simulink library "lib_transmission"  (Simulink 4.1.1)
undefined symbols (not defined in the file or in its folder): fc_map_spd, fc_max_trq, fc_spd_scale, fc_trq_scale, fd_inertia, fd_loss, fd_ratio, gb_inertia, gb_loss_const, gb_loss_input_spd_coeff, gb_loss_input_trq_coeff, gb_loss_output_spd_coeff, gb_loss_output_trq_coeff, gb_map_spd_out, gb_map_trq_in, gb_map_trq_out, gb_ratio, gb_spd_scale, gb_trq_scale, htc_inertia, htc_k_adv, htc_k_adv_coast, htc_max_coast_tr, htc_min_coast_tr, htc_sr, htc_sr_coast, htc_tr, htc_tr_coast, mc_map_spd, mc_max_trq, mc_overtrq_factor, mc_spd_scale, mc_trq_scale, tc_loss, tc_mc_to_fc_ratio, tx_eff_map, tx_map_spd, tx_map_trq, tx_pg_r, tx_pg_s, vc_idle_spd, vc_launch_spd
libraries: lib_transmission x2
(part 3 of 3)

== system lib_transmission/CVT gearbox  <gb>/loss (Nm)/Input Torque: 3-D interpolation ==
  output torque (N*m) : Inport  Port=1  LatchInput=off
  output speed (rad/s) : Inport  Port=2  LatchInput=off
  pulley ratio : Inport  Port=3  LatchInput=off
  Constant3 : Constant  Value=eps
  Constant4 : Constant  Value=0
  Demux2 : Demux  Outputs=2  BusSelectionMode=off
  Look-Up Table1 : Lookup  InputValues=[1:max(size(gb_ratio))]  OutputValues=gb_ratio
  Look-Up Table2 : Lookup  InputValues=[1:max(size(gb_ratio))]  OutputValues=gb_ratio
  Mux1 : Mux  Inputs=4
      settings: DisplayOption=none
  Mux2 : Mux  Inputs=3
      settings: DisplayOption=none
  Mux3 : Mux  Inputs=2
      settings: DisplayOption=none
  Mux4 : Mux  Inputs=2
      settings: DisplayOption=none
  Mux7 : Mux  Inputs=4
      settings: DisplayOption=none
  Product1 : Product  Inputs=3  Multiplication=Element-wise(.*)  SaturateOnIntegerOverflow=on
  Product2 : Product  Inputs=*//  Multiplication=Element-wise(.*)  SaturateOnIntegerOverflow=on
  Sum2 : Sum  Inputs=2  SaturateOnIntegerOverflow=on
  Switch1 : Switch  Threshold=eps
  indices of nearest pulley ratios for which there exist maps : Subsystem
      settings: RTWFcnNameOpts=Auto  RTWFileNameOpts=Auto
  linear eqn for power : Fcn  Expr=u[5]*(u[6]-u[3])+u[1]
  slope for linear interp. : Fcn  Expr=(u[1]-u[2])/(u[3]-u[4]+eps)
  trq in  look-up : Subsystem  mask{P1=gb_map_spd_out*gb_spd_scale, P2=gb_map_trq_in*gb_trq_scale, P3=gb_map_trq_out*gb_trq_scale, P4=gb_ratio}
      mask prompts: P1 "Vector of output speeds"; P2 "Vector of input torques"; P3 "Table of output torques"; P4 "Vector of gear ratios"
      settings: RTWFcnNameOpts=Auto  RTWFileNameOpts=Auto
  input torque (Nm) : Outport  Port=1  InitialOutput=0
  wires:
  pulley ratio/1 -> indices of nearest pulley ratios for which there exist maps/1(in_1), Mux2/3, Product2/3
  indices of nearest pulley ratios for which there exist maps/1(index of upper bounding map) -> Look-Up Table1/1, Mux7/3
  indices of nearest pulley ratios for which there exist maps/2(index of lower bounding map) -> Look-Up Table2/1, Mux7/4
  Mux7/1 -> trq in  look-up/1(In1)
  slope for linear interp./1 -> Mux2/2
  Mux2/1 -> linear eqn for power/1
  Mux1/1 -> Mux2/1, slope for linear interp./1
  Demux2/2 -> Mux1/2
  output torque (N*m)/1 -> Mux7/1
  Demux2/1 -> Mux1/1
  Look-Up Table1/1 -> Mux1/3, Mux3/1
  Look-Up Table2/1 -> Mux1/4, Mux3/2
  output speed (rad/s)/1 -> Mux7/2, Mux4/1, Mux4/2, Sum2/1, Switch1/2
  trq in  look-up/1(Out1) -> Product1/2
  Mux4/1 -> Product1/1
  Mux3/1 -> Product1/3
  Product1/1 -> Demux2/1
  linear eqn for power/1 -> Product2/1
  Sum2/1 -> Product2/2
  Product2/1 -> Switch1/1
  Switch1/1 -> input torque (Nm)/1
  Constant4/1 -> Switch1/3
  Constant3/1 -> Sum2/2

== system lib_transmission/SubLibraries/loss (Nm)/Block NOTES ==
  note: Revision Notes:
  note: 09/20/02:tm modifed lower input to switch after T_loss_at_input to pass the
      | total torque input as the loss when tx_eff=0
      | 5 July 2001:mpo changing loss block to a lookup table methodology
      | 12/20/00:tm revised loss saturation block. lower limit changed
      | from 1 to 0 and upper limit changed from 100 to inf to prevent over or under penalties

== system lib_transmission/SubLibraries/loss (Nm) old methodology/Block NOTES ==
  note: Revision Notes:
  note: 12/20/00:tm revised loss saturation block. lower limit changed
      | from 1 to 0 and upper limit changed from 100 to inf to prevent over or under penalties

== system lib_transmission/gearbox <gb>/Pout/Pin, neglecting inertia/Pout/Pin (neglecting inertia) ==
  in_1 : Inport  Port=1  LatchInput=off
  in_2 : Inport  Port=2  LatchInput=off
  Fcn : Fcn  Expr=1/u
  Product : Product  Inputs=2  Multiplication=Element-wise(.*)  SaturateOnIntegerOverflow=on
  out_1 : Outport  Port=1  InitialOutput=0
  wires:
  in_2/1 -> Fcn/1
  Product/1 -> out_1/1
  Fcn/1 -> Product/2
  in_1/1 -> Product/1

== system lib_transmission/gearbox <gb>/Pout/Pin, neglecting inertia/make division bombproof ==
  note: only add eps if Tin-Tinertia is == 0 (this avoids problems when Tin-Tineratia == -eps
      | which happens from time to time
  Tin-Tinertia : Inport  Port=1  LatchInput=off
  Block NOTES : Subsystem
      settings: RTWFcnNameOpts=Auto  RTWFileNameOpts=Auto
      mask Display: disp('Block\nNOTES')
  Constant : Constant  Orientation=up  Value=eps
  Constant1 : Constant  Orientation=up  Value=0
  Product : Product  Inputs=2  Multiplication=Element-wise(.*)  SaturateOnIntegerOverflow=on
  Relational Operator1 : RelationalOperator  Operator===
  make division bombproof : Sum  Inputs=++  SaturateOnIntegerOverflow=on
  Out1 : Outport  Port=1
  wires:
  make division bombproof/1 -> Out1/1
  Constant/1 -> Product/2
  Relational Operator1/1 -> Product/1
  Product/1 -> make division bombproof/2
  Constant1/1 -> Relational Operator1/2
  Tin-Tinertia/1 -> Relational Operator1/1, make division bombproof/1

== system lib_transmission/hydraulic torque converter <htc>/SR/K_adv ==
  "Req'd output trq and spd (Nm), (rad/s)" : Inport  Port=1  LatchInput=off
  >0 : Saturate  UpperLimit=inf  LowerLimit=eps  LinearizeAsGain=on
  K_adv=wout/(Tout)^0.5 : Fcn  Expr=u[2]/u[1]^0.5
  Saturation : Saturate  UpperLimit=max(htc_k_adv)  LowerLimit=min(htc_k_adv)  LinearizeAsGain=on
  K_adv : Outport  Port=1
  wires:
  >0/1 -> K_adv=wout/(Tout)^0.5/1
  "Req'd output trq and spd (Nm), (rad/s)"/1 -> >0/1
  K_adv=wout/(Tout)^0.5/1 -> Saturation/1
  Saturation/1 -> K_adv/1

== system lib_transmission/hydraulic torque converter <htc>/SR/K_adv_coast ==
  "Req'd output trq and spd (Nm), (rad/s)" : Inport  Port=1  LatchInput=off
  K_adv=wout/(abs(Tout))^0.5 : Fcn  Expr=u[2]/abs(u[1]+eps)^0.5
  Saturation : Saturate  UpperLimit=max(htc_k_adv_coast)  LowerLimit=min(htc_k_adv_coast)  LinearizeAsGain=on
  K_adv_coast : Outport  Port=1
  wires:
  K_adv=wout/(abs(Tout))^0.5/1 -> Saturation/1
  Saturation/1 -> K_adv_coast/1
  "Req'd output trq and spd (Nm), (rad/s)"/1 -> K_adv=wout/(abs(Tout))^0.5/1

== system lib_transmission/hydraulic torque converter <htc>/SR/shifting SR ==
  T,w req out : Inport  Port=1  LatchInput=off
  w in : Inport  Port=2  LatchInput=off
  SR : Inport  Port=3  LatchInput=off
  -3200 rpm/second allowable in engine speed : Gain  Gain=-3200*pi/30  Multiplication=Element-wise(K.*u)  SaturateOnIntegerOverflow=on
  >0 : Saturate  UpperLimit=inf  LowerLimit=eps  LinearizeAsGain=on
  Clock : Clock
      settings: DisplayTime=off  Decimation=10
  Memory3 : Memory  X0=eps  InheritSampleTime=off
      settings: RTWStateStorageClass=Auto
  Memory4 : Memory  X0=0  InheritSampleTime=off
      settings: RTWStateStorageClass=Auto
  MinMax : MinMax  Function=min  Inputs=2
  SRmax= wout/win,min : Product  Inputs=*/  Multiplication=Element-wise(.*)  SaturateOnIntegerOverflow=on
  dt=t-(t-1) : Sum  Inputs=+-  SaturateOnIntegerOverflow=on
  "shifting, then limit  engine speed change" : Switch  Threshold=eps
  win,min= win,prev+rate*dt : Sum  Inputs=++  SaturateOnIntegerOverflow=on
  wout,req : Selector  InputType=Vector  ElementSrc=Internal  Elements=2  RowSrc=Internal  Rows=1  ColumnSrc=Internal  Columns=1  InputPortWidth=2
  SR limited : Outport  Port=1  InitialOutput=0
  wires:
  -3200 rpm/second allowable in engine speed/1 -> win,min= win,prev+rate*dt/2
  >0/1 -> Memory3/1
  w in/1 -> >0/1
  MinMax/1 -> "shifting, then limit  engine speed change"/1
  "shifting, then limit  engine speed change"/1 -> SR limited/1
  SR/1 -> MinMax/2, "shifting, then limit  engine speed change"/3
  SRmax= wout/win,min/1 -> MinMax/1
  [shifting] -> "shifting, then limit  engine speed change"/2
  T,w req out/1 -> wout,req/1
  wout,req/1 -> SRmax= wout/win,min/1
  win,min= win,prev+rate*dt/1 -> SRmax= wout/win,min/2
  Memory3/1 -> win,min= win,prev+rate*dt/1
  dt=t-(t-1)/1 -> -3200 rpm/second allowable in engine speed/1
  Clock/1 -> dt=t-(t-1)/1, Memory4/1
  Memory4/1 -> dt=t-(t-1)/2

== system lib_transmission/hydraulic torque converter <htc>/T, shifting/T_max ==
  w_APU : Inport  Port=1  LatchInput=off
  TR : Inport  Port=2  LatchInput=off
  Saturation1 : Saturate  UpperLimit=max(fc_map_spd)*fc_spd_scale  LowerLimit=min(fc_map_spd)*fc_spd_scale  LinearizeAsGain=on
  Tin*TR= Tout : Product  Inputs=2  Multiplication=Element-wise(.*)  SaturateOnIntegerOverflow=on
  max_torque lookup : Lookup  InputValues=fc_map_spd*fc_spd_scale  OutputValues=fc_max_trq*fc_trq_scale
  T_max max gain from htc : Outport  Port=1  InitialOutput=0
  wires:
  max_torque lookup/1 -> Tin*TR= Tout/1
  TR/1 -> Tin*TR= Tout/2
  Tin*TR= Tout/1 -> T_max max gain from htc/1
  w_APU/1 -> Saturation1/1
  Saturation1/1 -> max_torque lookup/1

== system lib_transmission/hydraulic torque converter <htc>/T, shifting/engine speed estimator ==
  htc_spd_in_a : Inport  Port=1  LatchInput=off
  Memory2 : Memory  X0=0  InheritSampleTime=off
      settings: RTWStateStorageClass=Auto
  Out1 : Outport  Port=1
  wires:
  Memory2/1 -> Out1/1
  htc_spd_in_a/1 -> Memory2/1

== system lib_transmission/hydraulic torque converter for  parallel hybrid <htc>/SR/K_adv ==
  "Req'd output trq and spd (Nm), (rad/s)" : Inport  Port=1  LatchInput=off
  >0 : Saturate  UpperLimit=inf  LowerLimit=eps  LinearizeAsGain=on
  K_adv=wout/(Tout)^0.5 : Fcn  Expr=u[2]/u[1]^0.5
  Saturation : Saturate  UpperLimit=max(htc_k_adv)  LowerLimit=min(htc_k_adv)  LinearizeAsGain=on
  K_adv : Outport  Port=1
  wires:
  >0/1 -> K_adv=wout/(Tout)^0.5/1
  "Req'd output trq and spd (Nm), (rad/s)"/1 -> >0/1
  K_adv=wout/(Tout)^0.5/1 -> Saturation/1
  Saturation/1 -> K_adv/1

== system lib_transmission/hydraulic torque converter for  parallel hybrid <htc>/SR/K_adv_coast ==
  "Req'd output trq and spd (Nm), (rad/s)" : Inport  Port=1  LatchInput=off
  K_adv=wout/(abs(Tout))^0.5 : Fcn  Expr=u[2]/abs(u[1]+eps)^0.5
  Saturation : Saturate  UpperLimit=max(htc_k_adv_coast)  LowerLimit=0  LinearizeAsGain=on
  K_adv_coast : Outport  Port=1
  wires:
  K_adv=wout/(abs(Tout))^0.5/1 -> Saturation/1
  Saturation/1 -> K_adv_coast/1
  "Req'd output trq and spd (Nm), (rad/s)"/1 -> K_adv=wout/(abs(Tout))^0.5/1

== system lib_transmission/hydraulic torque converter for  parallel hybrid <htc>/SR/shifting SR ==
  T,w req out : Inport  Port=1  LatchInput=off
  w in : Inport  Port=2  LatchInput=off
  SR : Inport  Port=3  LatchInput=off
  -3200 rpm/second allowable in engine speed : Gain  Gain=-3200*pi/30  Multiplication=Element-wise(K.*u)  SaturateOnIntegerOverflow=on
  >0 : Saturate  UpperLimit=inf  LowerLimit=eps  LinearizeAsGain=on
  Clock : Clock
      settings: DisplayTime=off  Decimation=10
  Memory3 : Memory  X0=eps  InheritSampleTime=off
      settings: RTWStateStorageClass=Auto
  Memory4 : Memory  X0=0  InheritSampleTime=off
      settings: RTWStateStorageClass=Auto
  MinMax : MinMax  Function=min  Inputs=2
  SRmax= wout/win,min : Product  Inputs=*/  Multiplication=Element-wise(.*)  SaturateOnIntegerOverflow=on
  dt=t-(t-1) : Sum  Inputs=+-  SaturateOnIntegerOverflow=on
  "shifting, then limit  engine speed change" : Switch  Threshold=eps
  win,min= win,prev+rate*dt : Sum  Inputs=++  SaturateOnIntegerOverflow=on
  wout,req : Selector  InputType=Vector  ElementSrc=Internal  Elements=2  RowSrc=Internal  Rows=1  ColumnSrc=Internal  Columns=1  InputPortWidth=2
  SR limited : Outport  Port=1  InitialOutput=0
  wires:
  -3200 rpm/second allowable in engine speed/1 -> win,min= win,prev+rate*dt/2
  >0/1 -> Memory3/1
  w in/1 -> >0/1
  MinMax/1 -> "shifting, then limit  engine speed change"/1
  "shifting, then limit  engine speed change"/1 -> SR limited/1
  SR/1 -> MinMax/2, "shifting, then limit  engine speed change"/3
  SRmax= wout/win,min/1 -> MinMax/1
  [shifting] -> "shifting, then limit  engine speed change"/2
  T,w req out/1 -> wout,req/1
  wout,req/1 -> SRmax= wout/win,min/1
  win,min= win,prev+rate*dt/1 -> SRmax= wout/win,min/2
  Memory3/1 -> win,min= win,prev+rate*dt/1
  dt=t-(t-1)/1 -> -3200 rpm/second allowable in engine speed/1
  Clock/1 -> dt=t-(t-1)/1, Memory4/1
  Memory4/1 -> dt=t-(t-1)/2

== system lib_transmission/hydraulic torque converter for  parallel hybrid <htc>/T, shifting/T_max ==
  w_APU : Inport  Port=1  LatchInput=off
  TR : Inport  Port=2  LatchInput=off
  Block NOTES : Subsystem
      settings: RTWFcnNameOpts=Auto  RTWFileNameOpts=Auto
      mask Display: disp('Block\nNOTES')
  Constant : Constant  Value=1
  Gain : Gain  Gain=tc_mc_to_fc_ratio  Multiplication=Element-wise(K.*u)  SaturateOnIntegerOverflow=on
  Gain1 : Gain  Gain=tc_mc_to_fc_ratio  Multiplication=Element-wise(K.*u)  SaturateOnIntegerOverflow=on
  Saturation1 : Saturate  UpperLimit=max(fc_map_spd)*fc_spd_scale  LowerLimit=min(fc_map_spd)*fc_spd_scale  LinearizeAsGain=on
  Sum : Sum  Inputs=++  SaturateOnIntegerOverflow=on
  Switch : Switch  Threshold=eps
  Terminator : Terminator
  Tin*TR= Tout : Product  Inputs=2  Multiplication=Element-wise(.*)  SaturateOnIntegerOverflow=on
  max_torque  mc lookup1 : Lookup  InputValues=mc_map_spd*mc_spd_scale  OutputValues=mc_max_trq*mc_overtrq_factor*mc_trq_scale
  max_torque lookup : Lookup  InputValues=fc_map_spd*fc_spd_scale  OutputValues=fc_max_trq*fc_trq_scale
  T_max max gain from htc : Outport  Port=1  InitialOutput=0
  wires:
  [engine_on] -> Terminator/1
  Switch/1 -> Tin*TR= Tout/1
  Gain1/1 -> Switch/3, Sum/2
  Sum/1 -> Switch/1
  Constant/1 -> Switch/2
  max_torque  mc lookup1/1 -> Gain1/1
  Gain/1 -> max_torque  mc lookup1/1
  Saturation1/1 -> Gain/1, max_torque lookup/1
  max_torque lookup/1 -> Sum/1
  TR/1 -> Tin*TR= Tout/2
  Tin*TR= Tout/1 -> T_max max gain from htc/1
  w_APU/1 -> Saturation1/1

== system lib_transmission/hydraulic torque converter for  parallel hybrid <htc>/T, shifting/engine speed estimator ==
  htc_spd_in_a : Inport  Port=1  LatchInput=off
  Memory2 : Memory  X0=0  InheritSampleTime=off
      settings: RTWStateStorageClass=Auto
  Out1 : Outport  Port=1
  wires:
  Memory2/1 -> Out1/1
  htc_spd_in_a/1 -> Memory2/1

== system lib_transmission/CVT gearbox  <gb>/loss (Nm)/Input Torque: 3-D interpolation/indices of nearest pulley ratios for which there exist maps ==
  in_1 : Inport  Port=1  LatchInput=off
  Constant : Constant  Value=1
  Look-Up Table : Lookup  InputValues=fliplr(gb_ratio)  OutputValues=fliplr([1:max(size(gb_ratio))])
  Rounding Function : Rounding  Operator=fix
  Saturation : Saturate  UpperLimit=max(size(gb_ratio))  LowerLimit=1  LinearizeAsGain=on
  Sum : Sum  Inputs=++  SaturateOnIntegerOverflow=on
  index of upper bounding map : Outport  Port=1  InitialOutput=0
  index of lower bounding map : Outport  Port=2  InitialOutput=0
  wires:
  Look-Up Table/1 -> Rounding Function/1
  in_1/1 -> Look-Up Table/1
  Constant/1 -> Sum/1
  Rounding Function/1 -> Sum/2, index of lower bounding map/1
  Saturation/1 -> index of upper bounding map/1
  Sum/1 -> Saturation/1

== system lib_transmission/CVT gearbox  <gb>/loss (Nm)/Input Torque: 3-D interpolation/trq in  look-up ==
  In1 : Inport  Port=1  LatchInput=off
  S-Function5 : S-Function  FunctionName=sfun_gb_loss  Parameters=P1,P2,P3,P4  PortCounts=[]  SFunctionModules=''
  Out1 : Outport  Port=1  InitialOutput=0
  wires:
  S-Function5/1 -> Out1/1
  In1/1 -> S-Function5/1

== system lib_transmission/gearbox <gb>/Pout/Pin, neglecting inertia/make division bombproof/Block NOTES ==
  note: this block added 10 July 2001 by mpo:
      | originally a -eps was added to the denominator by default.
      | However, cases were ecountered where Tin-Tineratia was equal to -eps causing
      | the denominator to be zero. This added checking is more rhobust

== system lib_transmission/hydraulic torque converter for  parallel hybrid <htc>/T, shifting/T_max/Block NOTES ==
  note: Notes: engine_on flag causes algebric loop. Is it necessary?
      | Doesn't seem to be. Disabled 10/31/00:tm
